simulink model "getDataIMU6050_"  (R2020a)
settings: Solver=FixedStepDiscrete  StartTime=0.0  StopTime=1  FixedStep=1  RelTol=1e-3
settings Model: Creator=dangh  LastModifiedBy=dangh

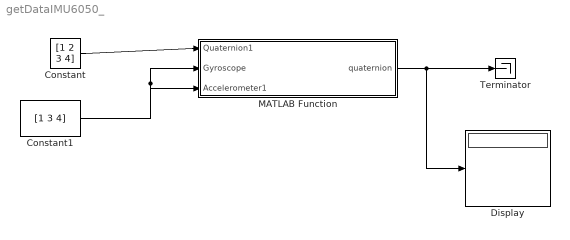
== system getDataIMU6050_ ==
  Constant : Constant  Value=[1 2 3 4]  OutDataTypeStr=double
  Constant1 : Constant  Value=[1 3 4]  OutDataTypeStr=double
  Display : Display
  MATLAB Function : MATLAB Function  TreatAsAtomicUnit=on
  Terminator : Terminator
  wires:
  Constant/1 -> MATLAB Function/1(Quaternion1)
  Constant1/1 -> MATLAB Function/3(Accelerometer1), MATLAB Function/2(Gyroscope)
  MATLAB Function/1(quaternion) -> Display/1, Terminator/1

== matlab function getDataIMU6050_/MATLAB Function ==
  data: Quaternion1 input; quaternion output; Gyroscope input; Accelerometer1 input
%function [residual, xhatOut] = EXTKALMAN(meas, deltat)
function quaternion  = UpdateIMU(Quaternion1, Gyroscope, Accelerometer1)

% Initialization
% persistent quaternion
% if isempty(quaternion)
%     quaternion = [1 0 0 0];     % output quaternion describing the Earth relative to the sensor
% end

SamplePeriod = 1/200;       %5ms
Beta = 0.1;               	% algorithm gain
q = [0 0 0 0];
%Accelerometer = [1 2 3]; 
Gyroscope = [1 2 3]; 

            q = Quaternion1; % short name local variable for readability
            Accelerometer = Accelerometer1;

            % Normalise accelerometer measurement
            if(norm(Accelerometer) == 0), return; end	% handle NaN
            Accelerometer = Accelerometer / norm(Accelerometer);	% normalise magnitude

            % Gradient decent algorithm corrective step
            F = [2*(q(2)*q(4) - q(1)*q(3)) - Accelerometer(1)
                2*(q(1)*q(2) + q(3)*q(4)) - Accelerometer(2)
                2*(0.5 - q(2)^2 - q(3)^2) - Accelerometer(3)];
            J = [-2*q(3),	2*q(4),    -2*q(1),	2*q(2)
                2*q(2),     2*q(1),     2*q(4),	2*q(3)
                0,         -4*q(2),    -4*q(3),	0    ];
            step = (J'*F);
            step = step / norm(step);	% normalise step magnitude

            % Compute rate of change of quaternion
            qDot = 0.5 * quaternProd1(q, [0 Gyroscope(1) Gyroscope(2) Gyroscope(3)]) - Beta * step';

            % Integrate to yield quaternion
            q = q + qDot * SamplePeriod;
            %Quaternion = q / norm(q); % normalise quaternion
            %q1 = q / norm(q); % normalise quaternion
            quaternion = q;
end
function ab = quaternProd1(a, b)
%QUATERNPROD Calculates the quaternion product
%
%   ab = quaternProd(a, b)
%
%   Calculates the quaternion product of quaternion a and b.
%
%   For more information see:
%   http://www.x-io.co.uk/node/8#quaternions
%
%	Date          Author          Notes
%	27/09/2011    SOH Madgwick    Initial release
    ab = zeros(1,4);
    ab(:,1) = a(:,1).*b(:,1)-a(:,2).*b(:,2)-a(:,3).*b(:,3)-a(:,4).*b(:,4);
    ab(:,2) = a(:,1).*b(:,2)+a(:,2).*b(:,1)+a(:,3).*b(:,4)-a(:,4).*b(:,3);
    ab(:,3) = a(:,1).*b(:,3)-a(:,2).*b(:,4)+a(:,3).*b(:,1)+a(:,4).*b(:,2);
    ab(:,4) = a(:,1).*b(:,4)+a(:,2).*b(:,3)-a(:,3).*b(:,2)+a(:,4).*b(:,1);
end
